simulink model "Day10"  (R2024b)
settings: Solver=VariableStepAuto  StartTime=0.0  StopTime=10.0  RelTol=1e-3
settings Model: Creator=jun_mac  LastModifiedBy=jun_mac

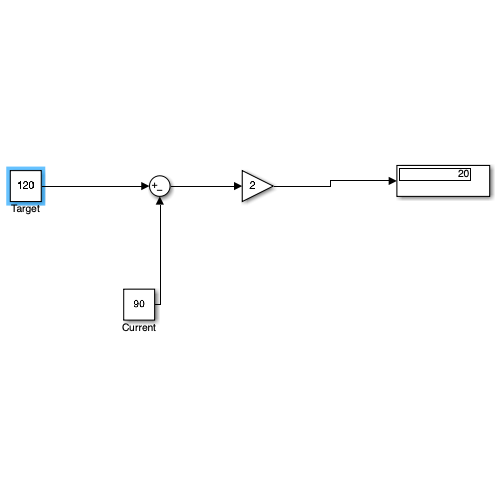
[thumbnail: Simulink's stored preview of the top-level diagram]
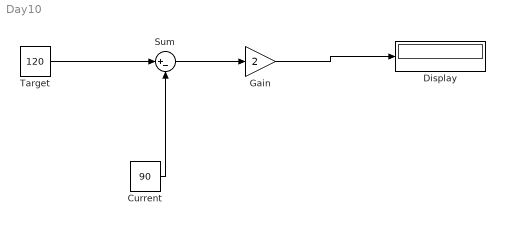
== system Day10 ==
  Current : Constant  Value=90
  Display : Display
  Gain : Gain  Gain=2
  Sum : Sum  Inputs=|+-
  Target : Constant  Value=120
  wires:
  Current/1 -> Sum/2
  Target/1 -> Sum/1
  Sum/1 -> Gain/1
  Gain/1 -> Display/1
